simulink model "lin_3dof_surface_vessel_model_w_estimated_states_2021"  (R2021b)
settings: Solver=VariableStepAuto  StartTime=0.0  StopTime=10
InitFcn:
  | % Rigid body
  | m = 127.92;
  | I_z = 61.967;
  | x_g = 0;
  | 
  | % Added mass
  | X_du = 3.262;
  | Y_dv = 28.89;
  | Y_dr = 0.525;
  | N_dv = 0.157;
  | N_dr = 13.98;
  | 
  | % Linear drag coefficients
  | X_u = -2.332;
  | Y_v = -4.673;
  | N_r = -0.01675;
  | Y_r = 0;
  | N_v = 0;
  | 
  | M = [m-X_du 0 0;
  |     0 m-Y_dv m*x_g-Y_dr;
  |     0 m*x_g-Y_dr I_z-N_dr];
  | 
  | D = [X_u 0 0;
  |     0 Y_v Y_r;
  |     0 N_v N_r];
  | 
  | eta_0 = [0.8; 0.2; 0];
  | 
  | lambda = 10;
settings Model: Creator=olegborisov  LastModifiedBy=mluser
settings SolverCC: AlgebraicLoopSolver=TrustRegion
settings DataIOCC: ReturnWorkspaceOutputs=off

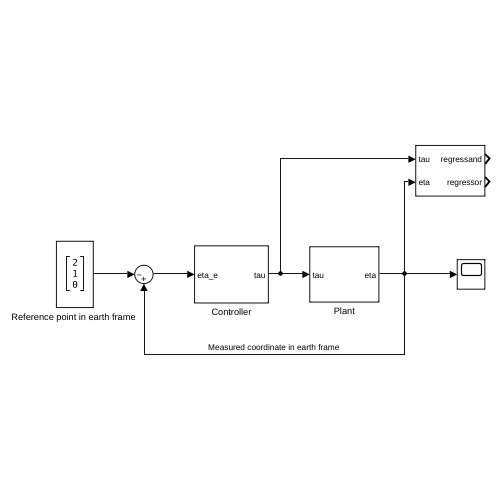
[thumbnail: Simulink's stored preview of the top-level diagram]
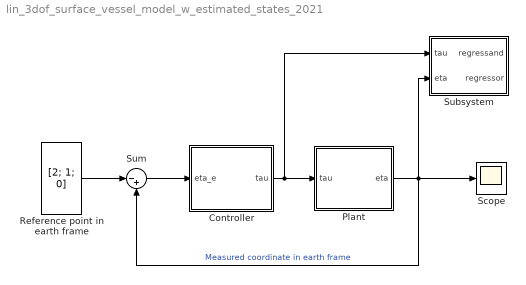
== system lin_3dof_surface_vessel_model_w_estimated_states_2021 ==
  Controller : Subsystem
  Plant : Subsystem
  "Reference point in earth frame " : Constant  Value=[2; 1; 0]  VectorParams1D=off
  Scope : Scope
  Subsystem : Subsystem
  Sum : Sum  Inputs=|-+
  wires:
  Plant/1(eta) -> Subsystem/2(eta), Scope/1, Sum/2  "Measured coordinate in earth frame"
  "Reference point in earth frame "/1 -> Sum/1
  Controller/1(tau) -> Subsystem/1(tau), Plant/1(tau)
  Sum/1 -> Controller/1(eta_e)

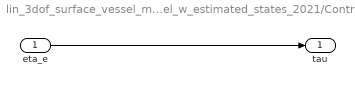
== system lin_3dof_surface_vessel_model_w_estimated_states_2021/Controller ==
  eta_e : Inport
  tau : Outport
  wires:
  eta_e/1 -> tau/1

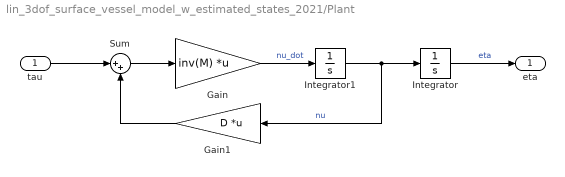
== system lin_3dof_surface_vessel_model_w_estimated_states_2021/Plant ==
  tau : Inport
  Gain : Gain  Gain=inv(M)  Multiplication=Matrix(K*u) (u vector)
  Gain1 : Gain  Gain=D  Multiplication=Matrix(K*u) (u vector)
  Integrator : Integrator  InitialCondition=eta_0
  Integrator1 : Integrator
  Sum : Sum  Inputs=|++
  eta : Outport
  wires:
  Integrator1/1 -> Integrator/1, Gain1/1  "nu"
  Gain/1 -> Integrator1/1  "nu_dot"
  Sum/1 -> Gain/1
  tau/1 -> Sum/1
  Gain1/1 -> Sum/2
  Integrator/1 -> eta/1  "eta"

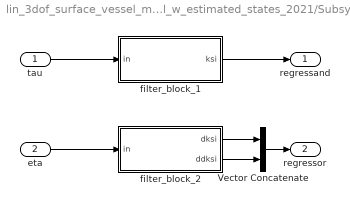
== system lin_3dof_surface_vessel_model_w_estimated_states_2021/Subsystem ==
  tau : Inport
  eta : Inport  Port=2
  Vector Concatenate : Concatenate  Mode=Multidimensional array
  filter_block_1 : Subsystem
  filter_block_2 : Subsystem
  regressand : Outport
  regressor : Outport  Port=2
  wires:
  tau/1 -> filter_block_1/1(in)
  filter_block_1/1(ksi) -> regressand/1
  eta/1 -> filter_block_2/1(in)
  filter_block_2/1(dksi) -> Vector Concatenate/1
  filter_block_2/2(ddksi) -> Vector Concatenate/2
  Vector Concatenate/1 -> regressor/1

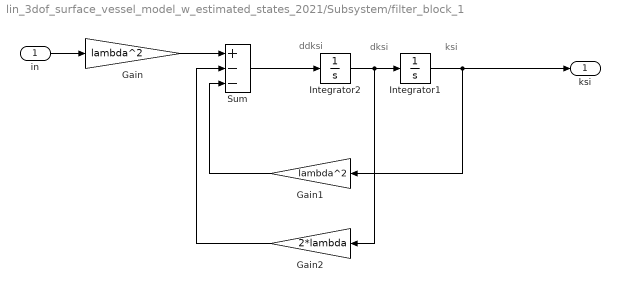
== system lin_3dof_surface_vessel_model_w_estimated_states_2021/Subsystem/filter_block_1 ==
  note: ksi
  note: dksi
  note: ddksi
  in : Inport
  Gain : Gain  Gain=lambda^2
  Gain1 : Gain  Gain=lambda^2
  Gain2 : Gain  Gain=2*lambda
  Integrator1 : Integrator
  Integrator2 : Integrator
  Sum : Sum  Inputs=+--
  ksi : Outport  VectorParamsAs1DForOutWhenUnconnected=off
  wires:
  Gain2/1 -> Sum/2
  Gain1/1 -> Sum/3
  Sum/1 -> Integrator2/1
  Gain/1 -> Sum/1
  Integrator1/1 -> ksi/1, Gain1/1
  Integrator2/1 -> Integrator1/1, Gain2/1
  in/1 -> Gain/1

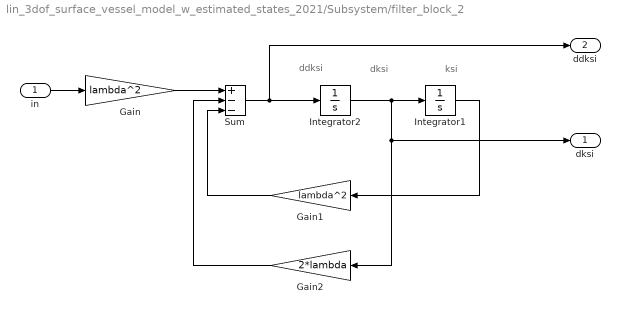
== system lin_3dof_surface_vessel_model_w_estimated_states_2021/Subsystem/filter_block_2 ==
  note: ddksi
  note: dksi
  note: ksi
  in : Inport
  Gain : Gain  Gain=lambda^2
  Gain1 : Gain  Gain=lambda^2
  Gain2 : Gain  Gain=2*lambda
  Integrator1 : Integrator
  Integrator2 : Integrator
  Sum : Sum  Inputs=+--
  dksi : Outport  VectorParamsAs1DForOutWhenUnconnected=off
  ddksi : Outport  Port=2  VectorParamsAs1DForOutWhenUnconnected=off
  wires:
  in/1 -> Gain/1
  Integrator2/1 -> Integrator1/1, dksi/1, Gain2/1
  Integrator1/1 -> Gain1/1
  Gain/1 -> Sum/1
  Sum/1 -> ddksi/1, Integrator2/1
  Gain1/1 -> Sum/3
  Gain2/1 -> Sum/2
